simulink model "HVACTestHarness"  (R2024b)
settings: Solver=daessc  StartTime=0  StopTime=50  RelTol=1e-3
PreLoadFcn:
  | % Load all parameters
  | HVACTestHarnessParams
undefined symbols (not defined in the file or in its folder): vehicleThermal
libraries: slpidlib x3, fl_lib x1, nesl_utility x1, ee_lib x1
Description:
  | Copyright 2022 - 2023 The MathWorks, Inc.
settings Model: PauseTimes=120  Creator=jjha  LastModifiedBy=jjha
settings SolverCC: ZeroCrossAlgorithm=Adaptive  DecoupledContinuousIntegration=on
settings DataIOCC: Decimation=10  ReturnWorkspaceOutputsName=SimlogBEVdata
settings OptimizationCC: ReuseModelBlockBuffer=off
settings DebuggingCC: IgnoredZcDiagnostic=none
settings RTWCC: GPUComputeCapability=3.5
settings SimscapeCC: SimscapeLogType=all  SimscapeLogSimulationStatistics=on  SimscapeLogName=simlogBEVsystemModel  SimscapeLogDecimation=10  SimscapeLogLimitData=off

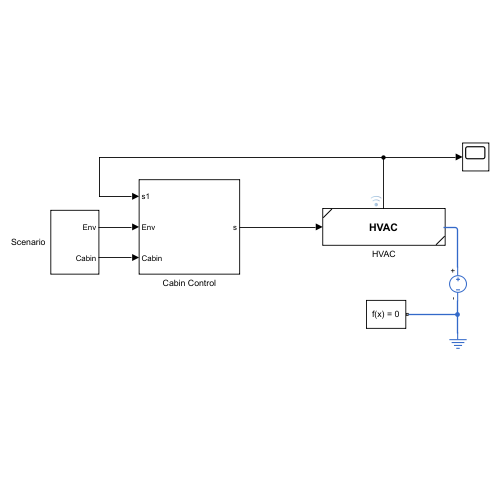
[thumbnail: Simulink's stored preview of the top-level diagram]
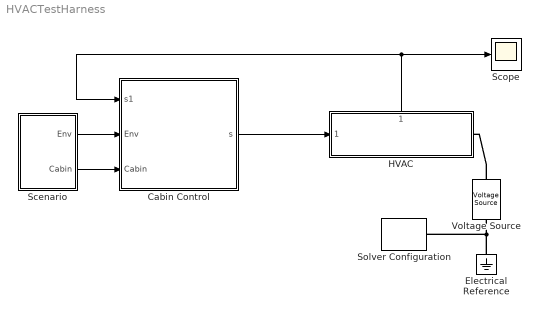
== system HVACTestHarness ==
  Cabin Control : Subsystem
  Electrical Reference : fl_lib/Electrical/Electrical Elements/Electrical Reference
  HVAC : Subsystem  ReferencedSubsystem=HVACEmpiricalRef
      settings: PortSchema="{\"entries\":[{\"content\":{\"sides\":[{\"content\":{\"connectorIds\":[\"In1\"]},\"type\":\"ConnectorPlacement.EquallySpacedRectSide\",\"uuid\":\"1deba8c1-465f-4d58-bbc9-ab0d1db98c17\"},{\"content\":{\"connectorIds\":[\"LConn1\"],\"side\":\"RIGHT\"},\"type\":\"ConnectorPlacement.EquallySpacedRectSide\",\"uuid\":\"8fbb44ad-e027-4231-94f3-f26435b888cd\"},{\"content\":{\"connectorIds\":[\"Out1\"],\"side\":\"TOP\"},\"type\":\"ConnectorPlacement.EquallySpacedRectSide\",\"uuid\":\"a2240e6e-7d5d-4f53-ba77-359aeea7e37b\"},{\"content\":{\"side\":\"BOTTOM\"},\"type\":\"ConnectorPlacement.EquallySpacedRectSide\",\"uuid\":\"1147aeee-559f-410b-9877-eca1e40225bf\"}]},\"type\":\"ConnectorPlacement.EquallySpacedConnector\",\"uuid\":\"aa6014e3-1db3-4f95-a470-f9bee2889440\"}],\"packageUris\":[\"http://schema.mathworks.com/mf0/Connector/R2020b\"],\"version\":\"1.0\"}"
  Scenario : Subsystem  Tag=cold weather
      settings: PortSchema="{\"entries\":[{\"content\":{\"sides\":[{\"content\":{\"connectorIds\":[]},\"type\":\"ConnectorPlacement.EquallySpacedRectSide\",\"uuid\":\"eb8d1f37-8208-4a35-a227-ee3e7712aac0\"},{\"content\":{\"connectorIds\":[],\"side\":\"RIGHT\"},\"type\":\"ConnectorPlacement.EquallySpacedRectSide\",\"uuid\":\"04c1ce39-a668-46a3-bb9a-590d9fa6d188\"},{\"content\":{\"connectorIds\":[\"Out1\",\"Out2\"],\"side\":\"TOP\"},\"type\":\"ConnectorPlacement.EquallySpacedRectSide\",\"uuid\":\"9d96e5e2-2b9d-42e1-9359-7f2aa762ed32\"}]},\"type\":\"ConnectorPlacement.EquallySpacedConnector\",\"uuid\":\"d1c4a0ed-0ab9-4caa-880d-25dbcbc152ad\"}],\"packageUris\":[\"http://schema.mathworks.com/mf0/Connector/R2020b\"],\"version\":\"1.0\"}"
  Scope : Scope
  Solver Configuration : nesl_utility/Solver Configuration  PhysicalDomain=network_engine_domain  SubClassName=solver  LeftPortType=input  RightPortType=generic  Tones=[]  Harmonics=[]  SimulateNoise=off  Profile=off  UseLocalSampling=off  EnableSwitchedLinearOptims=on  FrequencyDomain=off  UseCCode=off  RelTol=0.001  AbsTol=0.001  MinStep=1e-09  ToWorkspace=off  RevertToSquareIcSolve=off  NumHomotopyIterations=100  PhasorMode=off  PhasorModeNumHarmonics=1  ConsistencySolver=NEWTON_XTOL_AFTER_FTOL  IndexReductionMethod=DerivativeReplacement  DoDC=off  ResidualTolerance=1e-09  ConsistencyTolSource=GLOBAL  ConsistencyAbsTol=0.001  ConsistencyRelTol=0.001  ConsistencyTolFactor=0.001  UseLocalSolver=off  LocalSolverChoice=NE_BACKWARD_EULER_ADVANCER  ResolveIndetEquations=on  FunctionEvalNumThread=1  LocalSolverSampleTime=0.001  DoFixedCost=off  MaxNonlinIter=3  MaxModeIter=2  ComputeImpulses=off  ImpulseIterations=2  LinearAlgebra=auto  LinearAlgebraNumThread=0  EquationFormulation=NE_TIME_EF  DelaysMemoryBudget=1024  AutomaticFiltering=on  FilteringTimeConstant=0.001  PartitionStorageMethod=AS_NEEDED  PartitionMemoryBudget=1024  PartitionMethod=ROBUST  MultibodyUseLocalSolver=off  MultibodyLocalSolverChoice=ODE1  MultibodyLocalSolverSampleTime=0.001
  Voltage Source : ee_lib/Sources/Voltage Source  dc_voltage=0 V  ac_voltage=0 V  ac_shift=0 rad  ac_frequency=60 Hz  noise_mode=ee.enum.sources.noise.Disabled  PSD=0 V^2/Hz  sample_time=1e-3 s  repeatability=ee.enum.sources.repeatability.NotRepeatable  user_seed=0  auto_seed=3890346746  i_specify=off  i_priority=None  i=0 A  i_nominal_specify=off  i_nominal_value=1  i_nominal_unit=A  v_specify=off  v_priority=None  v=0 V  v_nominal_specify=off  v_nominal_value=1  v_nominal_unit=V
  wires:
  HVAC/1 -> Cabin Control/1(s1), Scope/1
  Scenario/2(Cabin) -> Cabin Control/3(Cabin)
  Cabin Control/1(s) -> HVAC/1
  Scenario/1(Env) -> Cabin Control/2(Env)
  connections:
  Voltage Source/LConn1 -- HVAC/LConn1
  Electrical Reference/LConn1 -- Solver Configuration/RConn1 -- Voltage Source/RConn1

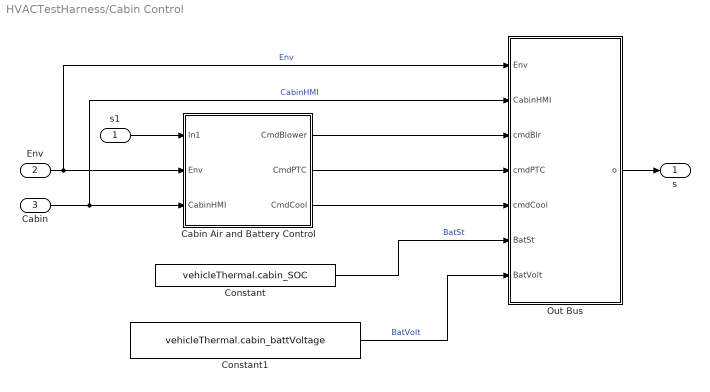
== system HVACTestHarness/Cabin Control ==
  s1 : Inport
  Env : Inport  Port=2
  Cabin : Inport  Port=3
  Cabin Air and Battery Control : Subsystem
  Constant : Constant  Value=vehicleThermal.cabin_SOC
  Constant1 : Constant  Value=vehicleThermal.cabin_battVoltage
  "Out Bus " : Subsystem
  s : Outport
  wires:
  Cabin/1 -> "Out Bus "/2(CabinHMI), Cabin Air and Battery Control/3(CabinHMI)  "CabinHMI"
  Env/1 -> Cabin Air and Battery Control/2(Env), "Out Bus "/1(Env)  "Env"
  s1/1 -> Cabin Air and Battery Control/1(In1)
  Cabin Air and Battery Control/1(CmdBlower) -> "Out Bus "/3(cmdBlr)
  Cabin Air and Battery Control/3(CmdCool) -> "Out Bus "/5(cmdCool)
  Constant/1 -> "Out Bus "/6(BatSt)  "BatSt"
  Constant1/1 -> "Out Bus "/7(BatVolt)  "BatVolt"
  "Out Bus "/1(o) -> s/1
  Cabin Air and Battery Control/2(CmdPTC) -> "Out Bus "/4(cmdPTC)

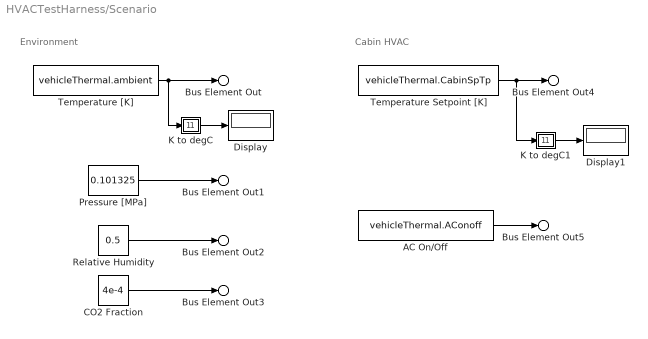
== system HVACTestHarness/Scenario ==
  note: Cabin HVAC
  note: Environment
  AC On/Off : Constant  Value=vehicleThermal.AConoff
  CO2 Fraction : Constant  Value=4e-4
  Display : Display
  Display1 : Display
  K to degC : Subsystem
  K to degC1 : Subsystem
  Pressure [MPa] : Constant  Value=0.101325
  Relative Humidity : Constant  Value=0.5
  Temperature Setpoint [K] : Constant  Value=vehicleThermal.CabinSpTp
  Temperature [K] : Constant  Value=vehicleThermal.ambient
  Bus Element Out : Outport  PortName=Env  Element=Tenv
  Bus Element Out1 : Outport  PortName=Env  Element=Penv
  Bus Element Out2 : Outport  PortName=Env  Element=RHenv
  Bus Element Out3 : Outport  PortName=Env  Element=CO2env
  Bus Element Out4 : Outport  Port=2  PortName=Cabin  Element=TpSetPoint
  Bus Element Out5 : Outport  Port=2  PortName=Cabin  Element=acOnOff
  wires:
  Relative Humidity/1 -> Bus Element Out2/1
  AC On/Off/1 -> Bus Element Out5/1
  Temperature Setpoint [K]/1 -> K to degC1/1(" "), Bus Element Out4/1
  CO2 Fraction/1 -> Bus Element Out3/1
  Temperature [K]/1 -> Bus Element Out/1, K to degC/1(" ")
  Pressure [MPa]/1 -> Bus Element Out1/1
  K to degC/1("  ") -> Display/1
  K to degC1/1("  ") -> Display1/1

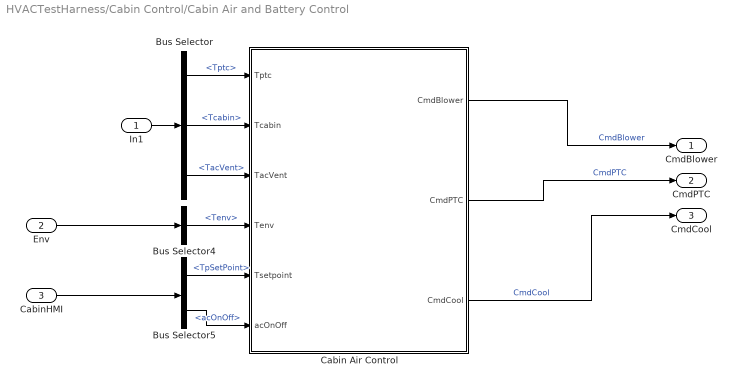
== system HVACTestHarness/Cabin Control/Cabin Air and Battery Control ==
  In1 : Inport
  Env : Inport  Port=2
  CabinHMI : Inport  Port=3
  Bus Selector : BusSelector  OutputSignals=Tptc,Tcabin,TacVent
  Bus Selector4 : BusSelector  OutputSignals=Tenv
  Bus Selector5 : BusSelector  OutputSignals=TpSetPoint,acOnOff
  Cabin Air Control : Subsystem
  CmdBlower : Outport
  CmdPTC : Outport  Port=2
  CmdCool : Outport  Port=3
  wires:
  Bus Selector5/2 -> Cabin Air Control/6(acOnOff)  "<acOnOff>"
  CabinHMI/1 -> Bus Selector5/1
  Bus Selector5/1 -> Cabin Air Control/5(Tsetpoint)  "<TpSetPoint>"
  Bus Selector/3 -> Cabin Air Control/3(TacVent)  "<TacVent>"
  Bus Selector/2 -> Cabin Air Control/2(Tcabin)  "<Tcabin>"
  Bus Selector/1 -> Cabin Air Control/1(Tptc)  "<Tptc>"
  Bus Selector4/1 -> Cabin Air Control/4(Tenv)  "<Tenv>"
  Cabin Air Control/1(CmdBlower) -> CmdBlower/1  "CmdBlower"
  Cabin Air Control/3(CmdCool) -> CmdCool/1  "CmdCool"
  In1/1 -> Bus Selector/1
  Env/1 -> Bus Selector4/1
  Cabin Air Control/2(CmdPTC) -> CmdPTC/1  "CmdPTC"

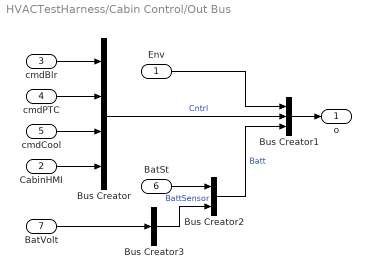
== system HVACTestHarness/Cabin Control/Out Bus  ==
  Env : Inport
  CabinHMI : Inport  Port=2
  cmdBlr : Inport  Port=3
  cmdPTC : Inport  Port=4
  cmdCool : Inport  Port=5
  BatSt : Inport  Port=6
  BatVolt : Inport  Port=7
  Bus Creator : BusCreator  Inputs=4
  Bus Creator1 : BusCreator  Inputs=3
  Bus Creator2 : BusCreator  Inputs=2
  Bus Creator3 : BusCreator  Inputs=1
  o : Outport
  wires:
  Bus Creator2/1 -> Bus Creator1/3  "Batt"
  Bus Creator3/1 -> Bus Creator2/2  "BattSensor"
  Bus Creator/1 -> Bus Creator1/2  "Cntrl"
  BatSt/1 -> Bus Creator2/1
  CabinHMI/1 -> Bus Creator/4
  Bus Creator1/1 -> o/1
  BatVolt/1 -> Bus Creator3/1
  Env/1 -> Bus Creator1/1
  cmdPTC/1 -> Bus Creator/2
  cmdCool/1 -> Bus Creator/3
  cmdBlr/1 -> Bus Creator/1

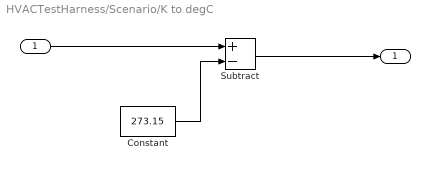
== system HVACTestHarness/Scenario/K to degC ==
  " " : Inport
  Constant : Constant  Value=273.15
  Subtract : Sum  Inputs=+-
  "  " : Outport
  wires:
  Constant/1 -> Subtract/2
  Subtract/1 -> "  "/1
  " "/1 -> Subtract/1

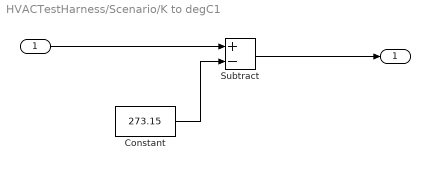
== system HVACTestHarness/Scenario/K to degC1 ==
  " " : Inport
  Constant : Constant  Value=273.15
  Subtract : Sum  Inputs=+-
  "  " : Outport
  wires:
  Constant/1 -> Subtract/2
  Subtract/1 -> "  "/1
  " "/1 -> Subtract/1

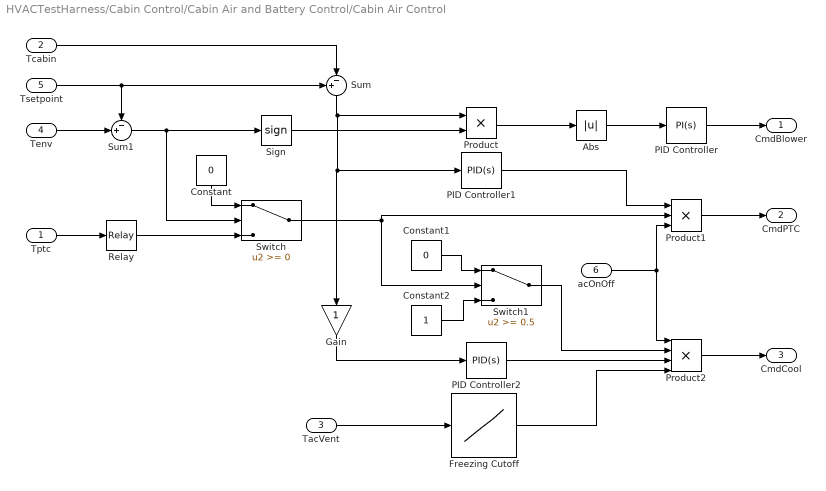
== system HVACTestHarness/Cabin Control/Cabin Air and Battery Control/Cabin Air Control ==
  Tptc : Inport
  Tcabin : Inport  Port=2
  TacVent : Inport  Port=3
  Tenv : Inport  Port=4
  Tsetpoint : Inport  Port=5
  acOnOff : Inport  Port=6
  Abs : Abs  SaturateOnIntegerOverflow=off
  Constant : Constant  Value=0
  Constant1 : Constant  Value=0
  Constant2 : Constant
  Freezing Cutoff : Lookup_n-D  NumberOfTableDimensions=1  BreakpointsForDimension1=[5 7 12 15]+273.15  IndexSearchMethod=Linear search  BeginIndexSearchUsingPreviousIndexResult=on  Table=[0 0 1 1]  InternalRulePriority=Speed  RndMeth=Simplest
  Gain : Gain
  PID Controller : slpidlib/PID Controller  Controller=PI  Form=Ideal  TimeDomain=Continuous-time  UseExternalTs=off  SampleTime=-1  IntegratorMethod=Forward Euler  FilterMethod=Forward Euler  ControllerParametersSource=internal  P=100  I=0.806408389739391  UseKiTs=off  D=0  UseExternalDerivativeSource=off  N=100  UseFilter=on  TunerSelectOption=Transfer Function Based (PID Tuner App)  ZeroCross=off  InitialConditionSource=internal  InitialConditionForIntegrator=0  InitialConditionForFilter=0  DifferentiatorICPrevScaledInput=0  ExternalReset=none  TrackingMode=off  Kt=1  LimitOutput=on  SatLimitsSource=internal  UpperSaturationLimit=1  LowerSaturationLimit=0  LinearizeAsGain=on  AntiWindupMode=back-calculation  Kb=1  LimitIntegrator=off  UpperIntegratorSaturationLimit=inf  LowerIntegratorSaturationLimit=-inf  POutMin=[]  POutMax=[]  IOutMin=[]  IOutMax=[]  DOutMin=[]  DOutMax=[]  NOutMin=[]  NOutMax=[]  SumOutMin=[]  SumOutMax=[]  SaturationOutMin=[]  SaturationOutMax=[]  PParamMin=[]  PParamMax=[]  IParamMin=[]  IParamMax=[]  DParamMin=[]  DParamMax=[]  NParamMin=[]  NParamMax=[]  KbParamMin=[]  KbParamMax=[]  KtParamMin=[]  KtParamMax=[]  KbOutMin=[]  KbOutMax=[]  KtOutMin=[]  KtOutMax=[]  IntegratorOutMin=[]  IntegratorOutMax=[]  FilterOutMin=[]  FilterOutMax=[]  SumI1OutMin=[]  SumI1OutMax=[]  SumI2OutMin=[]  SumI2OutMax=[]  SumI3OutMin=[]  SumI3OutMax=[]  SumI4OutMin=[]  SumI4OutMax=[]  SumDOutMin=[]  SumDOutMax=[]  DifferentiatorOutMin=[]  DifferentiatorOutMax=[]  FilterDiffOutCoefMin=[]  FilterDiffOutCoefMax=[]  ReciprocalOutMin=[]  ReciprocalOutMax=[]  SumDenOutMin=[]  SumDenOutMax=[]  SumNumOutMin=[]  SumNumOutMax=[]  DivideOutMin=[]  DivideOutMax=[]  UdiffTsProdOutMin=[]  UdiffTsProdOutMax=[]  NTsProdOutMin=[]  NTsProdOutMax=[]  UintegralTsProdOutMin=[]  UintegralTsProdOutMax=[]  UngainTsProdOutMin=[]  UngainTsProdOutMax=[]  ClampingZeroOutDataTypeStr=Inherit: Inherit via back propagation  ClampingZeroOutMin=[]  ClampingZeroOutMax=[]  FilterDenConstantOutDataTypeStr=Inherit: Inherit via back propagation  FilterDenConstantOutMin=[]  FilterDenConstantOutMax=[]  PCopyOutDataTypeStr=Inherit: Inherit via back propagation  PCopyOutMin=[]  PCopyOutMax=[]  NCopyOutDataTypeStr=Inherit: Inherit via back propagation  NCopyOutMin=[]  NCopyOutMax=[]  IntegratorContinuousStateAttributes=''  IntegratorStateMustResolveToSignalObject=off  IntegratorRTWStateStorageClass=Auto  FilterContinuousStateAttributes=''  FilterStateMustResolveToSignalObject=off  FilterRTWStateStorageClass=Auto  ParallelPVariant=Passthrough  IdealPVariant=InternalParameters  IVariant=InternalParameters  DVariant=Disabled  IntegratorVariant=Continuous  SatVariant=Enabled  AWVariant=BackCalculation  PCopyVariant=Disabled  TRVariant=Disabled  FdbkBlocksVariant=Forward  IdealPFdbkVariant=Disabled  SatFdbkVariant=Disabled  DerivativeFilterVariant=Disabled  NVariant=Disabled  NCopyVariant=Disabled_SignalSpec  FilterICVariant=Disabled  IntegratorICVariant=InternalICs  ExternalResetVariant=Disabled  TRSumVariant=Passthrough  SumFdbkVariant=Disabled  SumVariant=Sum_PI  TsampFilterVariant=InternalTs  TsampNgainVariant=Passthrough  TsampIntegralVariant=Disabled_SignalSpec  ExternalSaturationOutDataTypeStr=Inherit: Same as second input  DerivativeSourceVariant=Disabled  PreIntVariant=InternalPreInt
  PID Controller1 : slpidlib/PID Controller  Controller=PID  Form=Parallel  TimeDomain=Continuous-time  UseExternalTs=off  SampleTime=-1  IntegratorMethod=Forward Euler  FilterMethod=Forward Euler  ControllerParametersSource=internal  P=4746.62937899736  I=0.0523084188526522  UseKiTs=off  D=-417  UseExternalDerivativeSource=off  N=0.03278  UseFilter=on  TunerSelectOption=Transfer Function Based (PID Tuner App)  ZeroCross=off  InitialConditionSource=internal  InitialConditionForIntegrator=0  InitialConditionForFilter=0  DifferentiatorICPrevScaledInput=0  ExternalReset=none  TrackingMode=off  Kt=1  LimitOutput=on  SatLimitsSource=internal  UpperSaturationLimit=2000  LowerSaturationLimit=0  LinearizeAsGain=off  AntiWindupMode=clamping  Kb=1  LimitIntegrator=off  UpperIntegratorSaturationLimit=500  LowerIntegratorSaturationLimit=-500  POutMin=[]  POutMax=[]  IOutMin=[]  IOutMax=[]  DOutMin=[]  DOutMax=[]  NOutMin=[]  NOutMax=[]  SumOutMin=[]  SumOutMax=[]  SaturationOutMin=[]  SaturationOutMax=[]  PParamMin=[]  PParamMax=[]  IParamMin=[]  IParamMax=[]  DParamMin=[]  DParamMax=[]  NParamMin=[]  NParamMax=[]  KbParamMin=[]  KbParamMax=[]  KtParamMin=[]  KtParamMax=[]  KbOutMin=[]  KbOutMax=[]  KtOutMin=[]  KtOutMax=[]  IntegratorOutMin=[]  IntegratorOutMax=[]  FilterOutMin=[]  FilterOutMax=[]  SumI1OutMin=[]  SumI1OutMax=[]  SumI2OutMin=[]  SumI2OutMax=[]  SumI3OutMin=[]  SumI3OutMax=[]  SumI4OutMin=[]  SumI4OutMax=[]  SumDOutMin=[]  SumDOutMax=[]  DifferentiatorOutMin=[]  DifferentiatorOutMax=[]  FilterDiffOutCoefMin=[]  FilterDiffOutCoefMax=[]  ReciprocalOutMin=[]  ReciprocalOutMax=[]  SumDenOutMin=[]  SumDenOutMax=[]  SumNumOutMin=[]  SumNumOutMax=[]  DivideOutMin=[]  DivideOutMax=[]  UdiffTsProdOutMin=[]  UdiffTsProdOutMax=[]  NTsProdOutMin=[]  NTsProdOutMax=[]  UintegralTsProdOutMin=[]  UintegralTsProdOutMax=[]  UngainTsProdOutMin=[]  UngainTsProdOutMax=[]  ClampingZeroOutDataTypeStr=Inherit: Inherit via back propagation  ClampingZeroOutMin=[]  ClampingZeroOutMax=[]  FilterDenConstantOutDataTypeStr=Inherit: Inherit via back propagation  FilterDenConstantOutMin=[]  FilterDenConstantOutMax=[]  PCopyOutDataTypeStr=Inherit: Inherit via back propagation  PCopyOutMin=[]  PCopyOutMax=[]  NCopyOutDataTypeStr=Inherit: Inherit via back propagation  NCopyOutMin=[]  NCopyOutMax=[]  IntegratorContinuousStateAttributes=''  IntegratorStateMustResolveToSignalObject=off  IntegratorRTWStateStorageClass=Auto  FilterContinuousStateAttributes=''  FilterStateMustResolveToSignalObject=off  FilterRTWStateStorageClass=Auto  ParallelPVariant=InternalParameters  IdealPVariant=Disabled  IVariant=InternalParameters  DVariant=InternalParameters  IntegratorVariant=Continuous  SatVariant=Enabled  AWVariant=ContClampingParallel  PCopyVariant=Disabled  TRVariant=Disabled  FdbkBlocksVariant=Forward  IdealPFdbkVariant=Disabled  SatFdbkVariant=Disabled  DerivativeFilterVariant=ContFilter  NVariant=InternalParameters  NCopyVariant=Disabled  FilterICVariant=InternalICsFilter  IntegratorICVariant=InternalICs  ExternalResetVariant=Disabled  TRSumVariant=Passthrough  SumFdbkVariant=Disabled  SumVariant=Sum_PID  TsampFilterVariant=InternalTs  TsampNgainVariant=Passthrough  TsampIntegralVariant=Disabled_SignalSpec  ExternalSaturationOutDataTypeStr=Inherit: Same as second input  DerivativeSourceVariant=ErrorSignal  PreIntVariant=InternalPreInt
  PID Controller2 : slpidlib/PID Controller  Controller=PID  Form=Parallel  TimeDomain=Continuous-time  UseExternalTs=off  SampleTime=-1  IntegratorMethod=Forward Euler  FilterMethod=Forward Euler  ControllerParametersSource=internal  P=1  I=2.6  UseKiTs=off  D=-417  UseExternalDerivativeSource=off  N=0.03278  UseFilter=on  TunerSelectOption=Transfer Function Based (PID Tuner App)  ZeroCross=off  InitialConditionSource=internal  InitialConditionForIntegrator=0  InitialConditionForFilter=0  DifferentiatorICPrevScaledInput=0  ExternalReset=none  TrackingMode=off  Kt=1  LimitOutput=on  SatLimitsSource=internal  UpperSaturationLimit=0  LowerSaturationLimit=-1500  LinearizeAsGain=off  AntiWindupMode=back-calculation  Kb=1  LimitIntegrator=off  UpperIntegratorSaturationLimit=500  LowerIntegratorSaturationLimit=-500  POutMin=[]  POutMax=[]  IOutMin=[]  IOutMax=[]  DOutMin=[]  DOutMax=[]  NOutMin=[]  NOutMax=[]  SumOutMin=[]  SumOutMax=[]  SaturationOutMin=[]  SaturationOutMax=[]  PParamMin=[]  PParamMax=[]  IParamMin=[]  IParamMax=[]  DParamMin=[]  DParamMax=[]  NParamMin=[]  NParamMax=[]  KbParamMin=[]  KbParamMax=[]  KtParamMin=[]  KtParamMax=[]  KbOutMin=[]  KbOutMax=[]  KtOutMin=[]  KtOutMax=[]  IntegratorOutMin=[]  IntegratorOutMax=[]  FilterOutMin=[]  FilterOutMax=[]  SumI1OutMin=[]  SumI1OutMax=[]  SumI2OutMin=[]  SumI2OutMax=[]  SumI3OutMin=[]  SumI3OutMax=[]  SumI4OutMin=[]  SumI4OutMax=[]  SumDOutMin=[]  SumDOutMax=[]  DifferentiatorOutMin=[]  DifferentiatorOutMax=[]  FilterDiffOutCoefMin=[]  FilterDiffOutCoefMax=[]  ReciprocalOutMin=[]  ReciprocalOutMax=[]  SumDenOutMin=[]  SumDenOutMax=[]  SumNumOutMin=[]  SumNumOutMax=[]  DivideOutMin=[]  DivideOutMax=[]  UdiffTsProdOutMin=[]  UdiffTsProdOutMax=[]  NTsProdOutMin=[]  NTsProdOutMax=[]  UintegralTsProdOutMin=[]  UintegralTsProdOutMax=[]  UngainTsProdOutMin=[]  UngainTsProdOutMax=[]  ClampingZeroOutDataTypeStr=Inherit: Inherit via back propagation  ClampingZeroOutMin=[]  ClampingZeroOutMax=[]  FilterDenConstantOutDataTypeStr=Inherit: Inherit via back propagation  FilterDenConstantOutMin=[]  FilterDenConstantOutMax=[]  PCopyOutDataTypeStr=Inherit: Inherit via back propagation  PCopyOutMin=[]  PCopyOutMax=[]  NCopyOutDataTypeStr=Inherit: Inherit via back propagation  NCopyOutMin=[]  NCopyOutMax=[]  IntegratorContinuousStateAttributes=''  IntegratorStateMustResolveToSignalObject=off  IntegratorRTWStateStorageClass=Auto  FilterContinuousStateAttributes=''  FilterStateMustResolveToSignalObject=off  FilterRTWStateStorageClass=Auto  ParallelPVariant=InternalParameters  IdealPVariant=Disabled  IVariant=InternalParameters  DVariant=InternalParameters  IntegratorVariant=Continuous  SatVariant=Enabled  AWVariant=BackCalculation  PCopyVariant=Disabled  TRVariant=Disabled  FdbkBlocksVariant=Forward  IdealPFdbkVariant=Disabled  SatFdbkVariant=Disabled  DerivativeFilterVariant=ContFilter  NVariant=InternalParameters  NCopyVariant=Disabled  FilterICVariant=InternalICsFilter  IntegratorICVariant=InternalICs  ExternalResetVariant=Disabled  TRSumVariant=Passthrough  SumFdbkVariant=Disabled  SumVariant=Sum_PID  TsampFilterVariant=InternalTs  TsampNgainVariant=Passthrough  TsampIntegralVariant=Disabled_SignalSpec  ExternalSaturationOutDataTypeStr=Inherit: Same as second input  DerivativeSourceVariant=ErrorSignal  PreIntVariant=InternalPreInt
  Product : Product
  Product1 : Product  Inputs=3
  Product2 : Product  Inputs=4
  Relay : Relay  OnSwitchValue=45+273.15  OffSwitchValue=35+273.15  OnOutputValue=0  OffOutputValue=1  ZeroCross=off
  Sign : Signum
  Sum : Sum  Inputs=+-|
  Sum1 : Sum  Inputs=-+|
  Switch : Switch  SaturateOnIntegerOverflow=off  InputSameDT=off
  Switch1 : Switch  Threshold=0.5  SaturateOnIntegerOverflow=off  InputSameDT=off
  CmdBlower : Outport
  CmdPTC : Outport  Port=2
  CmdCool : Outport  Port=3
  wires:
  Abs/1 -> PID Controller/1
  acOnOff/1 -> Product1/3, Product2/1
  TacVent/1 -> Freezing Cutoff/1
  Freezing Cutoff/1 -> Product2/4
  Gain/1 -> PID Controller2/1
  Constant2/1 -> Switch1/3
  Constant1/1 -> Switch1/1
  Switch1/1 -> Product2/2
  Product2/1 -> CmdCool/1
  PID Controller2/1 -> Product2/3
  Sum/1 -> Gain/1, PID Controller1/1, Product/1
  Product1/1 -> CmdPTC/1
  PID Controller1/1 -> Product1/1
  Tcabin/1 -> Sum/2
  Tptc/1 -> Relay/1
  Relay/1 -> Switch/3
  Switch/1 -> Switch1/2, Product1/2
  Constant/1 -> Switch/1
  Sign/1 -> Product/2
  Tenv/1 -> Sum1/2
  PID Controller/1 -> CmdBlower/1
  Product/1 -> Abs/1
  Sum1/1 -> Sign/1, Switch/2
  Tsetpoint/1 -> Sum/1, Sum1/1
